simulink model "balloon_sim_sol"  (R2023b)
settings: Solver=ode3  StartTime=0.0  StopTime=600  FixedStep=0.01  RelTol=1e-3
values from neighbouring files (symbols this model uses):
  A = [ -1 0 0 ; 0 0 1 ; 1 0 -1/2 ]    [balloon_par_sol.m]    (also in dmass_par_sol.m = [ 0 0 1 0 ; 0 0 0 1 ; -k/m1 k/m1 0 0 ; k/m2 -k/m2 0 0 ])
  a_vect = [ k ; d ; m ]    [MSD_par_sol.m]    (also in balloon_par_sol.m = -At(3,:)'; dmass_par_sol.m = -At(4,1:4)')
  alpha_vect = poly3traj([p0;v0],[pT;vT],H)    [MSD_par_sol.m]    (also in balloon_par_sol.m = poly5traj([h0;v0;a0],[hT;vT;aT],T); dmass_par_sol.m = poly7traj(z0,zT,H))
  B = [ 1 ; 0 ; 0 ]    [balloon_par_sol.m]    (also in dmass_par_sol.m = [ 0 ; 0 ; 1/m1 ; 0 ])
  C = [ 0 , 1 , 0 ]    [balloon_par_sol.m]
settings Model: Creator=jerome  LastModifiedBy=jerome
settings ModelReferenceCC: EnableRefExpFcnMdlSchedulingChecks=on

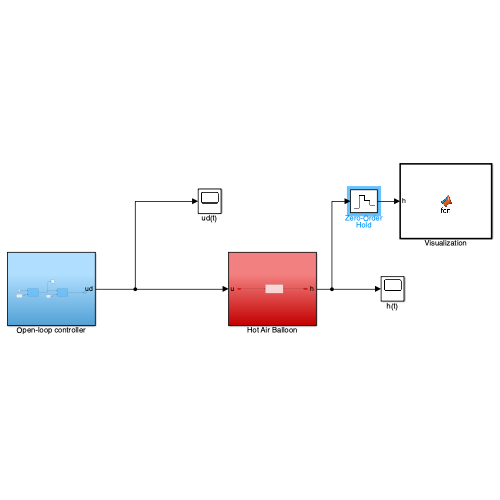
[thumbnail: Simulink's stored preview of the top-level diagram]
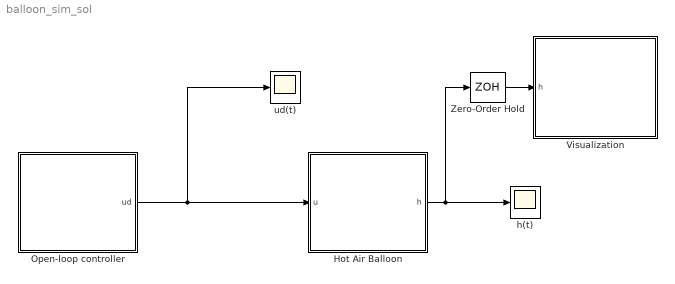
== system balloon_sim_sol ==
  Hot Air Balloon : Subsystem
  Open-loop controller : Subsystem
  Visualization : MATLAB Function  TreatAsAtomicUnit=on
  Zero-Order Hold : ZeroOrderHold  SampleTime=2
  h(t) : Scope
  ud(t) : Scope
  wires:
  Open-loop controller/1(ud) -> ud(t)/1, Hot Air Balloon/1(u)
  Hot Air Balloon/1(h) -> Zero-Order Hold/1, h(t)/1
  Zero-Order Hold/1 -> Visualization/1(h)

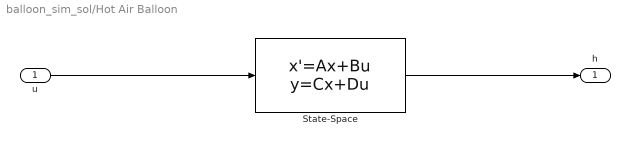
== system balloon_sim_sol/Hot Air Balloon ==
  u : Inport
  State-Space : StateSpace  A=A  B=B  C=C  D=0  InitialCondition=[0;0;0]
  h : Outport
  wires:
  State-Space/1 -> h/1
  u/1 -> State-Space/1

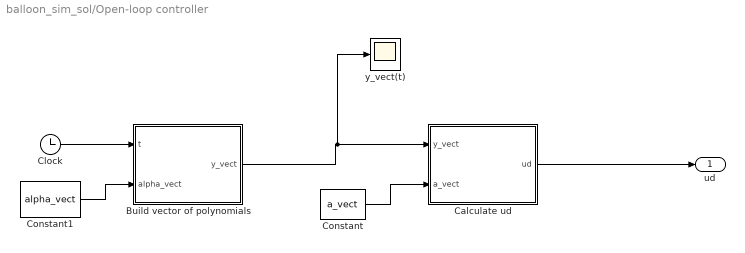
== system balloon_sim_sol/Open-loop controller ==
  Build vector of polynomials : MATLAB Function  TreatAsAtomicUnit=on
  Calculate ud : MATLAB Function  TreatAsAtomicUnit=on
  Clock : Clock
  Constant : Constant  Value=a_vect  VectorParams1D=off
  Constant1 : Constant  Value=alpha_vect  VectorParams1D=off
  y_vect(t) : Scope
  ud : Outport
  wires:
  Build vector of polynomials/1(y_vect) -> y_vect(t)/1, Calculate ud/1(y_vect)
  Constant/1 -> Calculate ud/2(a_vect)
  Constant1/1 -> Build vector of polynomials/2(alpha_vect)
  Clock/1 -> Build vector of polynomials/1(t)
  Calculate ud/1(ud) -> ud/1

== matlab function balloon_sim_sol/Open-loop controller/Build vector of polynomials ==
  data: t input; y_vect output; alpha_vect input
function y_vect = fcn(t,alpha_vect)


t_vect0 = [ 1 ; t ; t^2 ; t^3 ; t^4 ; t^5 ]; % vector of t values
t_vect1 = [ 0 ; 1 ; 2*t ; 3*t^2 ; 4*t^3 ; 5*t^4 ]; % derivative of t_vect0
t_vect2 = [ 0 ; 0 ; 2 ; 2*3*t ; 3*4*t^2 ; 4*5*t^3 ]; % derivative of t_vect1
t_vect3 = [ 0 ; 0 ; 0 ; 2*3 ; 2*3*4*t ; 3*4*5*t^2 ]; % derivative of t_vect2



yd = t_vect0'*alpha_vect;
yd_dot = t_vect1'*alpha_vect;
yd_ddot = t_vect2'*alpha_vect;
yd_3dot = t_vect3'*alpha_vect;

y_vect = [ yd ; yd_dot ; yd_ddot ; yd_3dot ];

== matlab function balloon_sim_sol/Open-loop controller/Calculate ud ==
  data: y_vect input; ud output; a_vect input
function ud = fcn(y_vect,a_vect)

ae_vect = [ a_vect ; 1 ];


% computation open-loop input
ud = ae_vect' * y_vect;

== matlab function balloon_sim_sol/Visualization ==
  data: h input
function fcn(h)

sf = 2.5; % scale factor
% balloon
    Xballoon = sf*[ 0 ; 0.6 ; 2.2 ; 3 ; 3 ; 2.2 ; 1.2 ; 0 ; -1.2 ; -2.2 ; -3 ; -3 ; -2.2 ; -0.6 ];
    Yballoon = sf*[ 1.2; 2; 3 ; 4 ; 5 ; 6; 6.4 ; 6.6 ; 6.4 ; 6 ; 5 ; 4 ; 3 ; 2 ]; 

% basket
    Xbasket = sf*[ 0.6 ; 0.6 ; -0.6 ; -0.6 ];
    Ybasket = sf*[ 0 ; 0.7 ; 0.7 ; 0 ];
    
% cables
    Xcable1 = sf*[ 0.6 ; 0.6 ];
    Ycable1 = sf*[ 0.7 ; 2 ];
    Xcable2 = sf*[ -0.6 ; -0.6 ];
    Ycable2 = sf*[ 0.7 ; 2 ];

    

% calculate graphical position of balloon
      PosXballoon = Xballoon;
      PosYballoon = Yballoon + h;

      PosXbasket = Xbasket;
      PosYbasket = Ybasket + h;

      PosXcable1 = Xcable1;
      PosYcable1 = Ycable1 + h;
      PosXcable2 = Xcable2;
      PosYcable2 = Ycable2 + h;

% to be able to use 'fill' even though the function is not supported for code generation
% see https://se.mathworks.com/help/simulink/slref/coder.extrinsic.html
coder.extrinsic('fill'); 

% draw the balloon
fill(PosXballoon,PosYballoon,'y');
hold on
brwn = [200 100 16]/256;
fill(PosXbasket,PosYbasket,brwn);
line(PosXcable1,PosYcable1,'Color','k','LineWidth',1);
line(PosXcable2,PosYcable2,'Color','k','LineWidth',1);
Xground = [-100;100];
Yground = [0;0];
Xgrass = [-100;-100;100;100];
Ygrass = [-20;0;0;-20];
line(Xground,Yground,'Color','k','LineWidth',3);
fill(Xgrass,Ygrass,'g');

hold off


axis([-60 60 -10 110]);
title('Open-loop control of a hot air balloon', 'FontSize',20);
axis square;
grid on;
lightBlue = [91, 207, 244] / 255;
set(gca,'Color',lightBlue);

drawnow;
